simulink model "final_proj_part_d"  (R2023b)
settings: Solver=ode45  StartTime=0.0  StopTime=10  RelTol=1e-3  EnableMultiTasking=on
libraries: roblocks x2
settings Model: Creator=Chris  LastModifiedBy=kangwang
settings SolverCC: AlgebraicLoopSolver=TrustRegion
settings DataIOCC: LimitDataPoints=on  SaveFormat=Array  SignalLoggingSaveFormat=ModelDataLogs  ReturnWorkspaceOutputs=off
settings OptimizationCC: InitFltsAndDblsToZero=on  LifeSpan=inf
settings DebuggingCC: SaveWithParameterizedLinksMsg=none  UnderspecifiedInitializationDetection=Classic  MergeDetectMultiDrivingBlocksExec=none  SignalResolutionControl=TryResolveAllWithWarning  SolverPrmCheckMsg=warning  MultiTaskDSMMsg=warning  MultiTaskCondExecSysMsg=none  UnconnectedInputMsg=warning  UnconnectedOutputMsg=warning  UnconnectedLineMsg=warning  SFUnexpectedBacktrackingDiag=warning  SFNoUnconditionalDefaultTransitionDiag=warning  SFExecutionAtInitializationDiag=none  ArithmeticOperatorsInVariantConditions=warning
settings HardwareCC: ProdBitPerPointer=32  ProdBitPerSizeT=32  ProdBitPerPtrDiffT=32  ProdLargestAtomicFloat=None  ProdIntDivRoundTo=Undefined  ProdEndianess=Unspecified  ProdWordSize=32  ProdHWDeviceType=32-bit Generic
settings ModelReferenceCC: PropagateSignalLabelsOutOfModel=off
settings SFSimCC: SimUseLocalCustomCode=off  CustomCodeUndefinedFunction=UseInterfaceOnly
settings RTWCC: RTWUseLocalCustomCode=off
settings CodeAppCC: StateflowObjectComments=on
settings GRTTargetCC: TargetFcnLib=ansi_tfl_tmw.mat  TargetLangStandard=C89/C90 (ANSI)  CombineOutputUpdateFcns=off  GRTInterface=on
settings ConfigComp: CovMetricSettings=dw  CovSaveCumulativeToWorkspaceVar=on  CovSaveSingleToWorkspaceVar=on  CovExternalEMLEnable=off

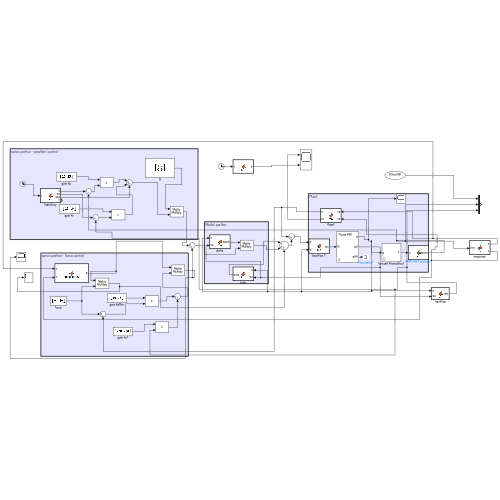
[thumbnail: Simulink's stored preview of the top-level diagram]
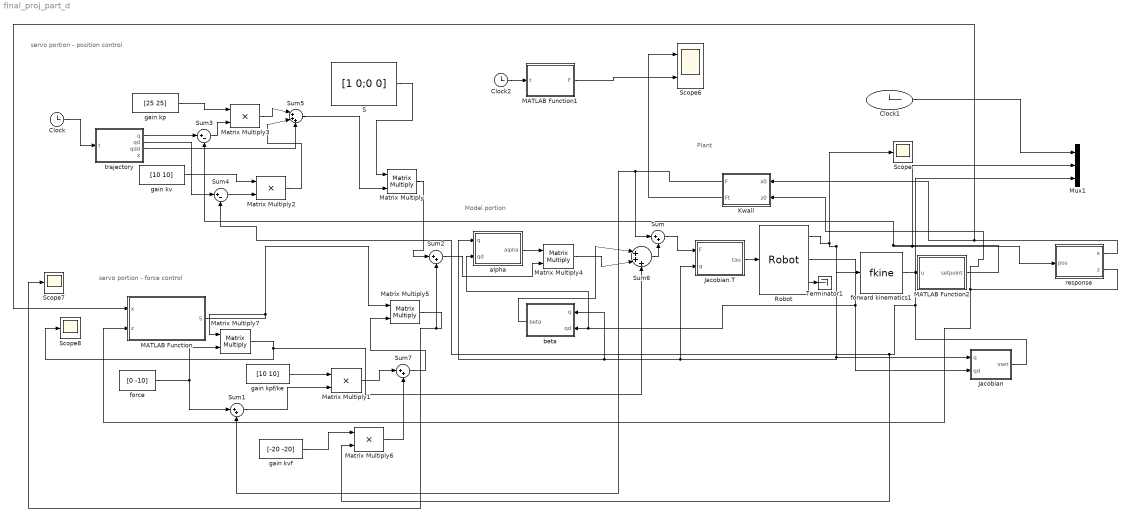
== system final_proj_part_d ==
  note: servo portion - force control
  note: Model portion
  note: Plant
  note: servo portion - position control
  Clock : Clock
  Clock1 : Clock
  Clock2 : Clock
  Jacobian : MATLAB Function  TreatAsAtomicUnit=on
  "Jacobian.T " : MATLAB Function  TreatAsAtomicUnit=on
  Kwall : MATLAB Function  TreatAsAtomicUnit=on
  MATLAB Function : MATLAB Function  TreatAsAtomicUnit=on
  MATLAB Function1 : MATLAB Function  TreatAsAtomicUnit=on
  MATLAB Function2 : MATLAB Function  TreatAsAtomicUnit=on
  Matrix Multiply{,4..5,7} (4 alike) : Product  Multiplication=Matrix(*)
  Matrix Multiply{1..3,6} (4 alike) : Product
  Mux1 : Mux  Inputs=3
  Robot : roblocks/Arm/Robot  robot=p560  q0=qn
  S : Constant  Value=[1 0;0 0]
  Scope : Scope
  Scope6 : Scope  NumInputPorts=2
  Scope7 : Scope
  Scope8 : Scope
  Sum{,1..2,7} (4 alike) : Sum  Inputs=|++
  Sum3 : Sum  Inputs=|+-
  Sum4 : Sum  Inputs=|+-
  Sum5 : Sum  Inputs=|+++
  Sum6 : Sum  Inputs=|+++
  Terminator1 : Terminator
  alpha : MATLAB Function  TreatAsAtomicUnit=on
  beta : MATLAB Function  TreatAsAtomicUnit=on
  force : Constant  Value=[0 -10]
  forward kinematics1 : roblocks/Arm/fkine  robot=robot
  gain kp : Constant  Value=[25 25]
  gain kpf/ke : Constant  Value=[10 10]
  gain kv : Constant  Value=[10 10]
  gain kvf : Constant  Value=[-20 -20]
  response : MATLAB Function  TreatAsAtomicUnit=on
  trajectory : MATLAB Function  TreatAsAtomicUnit=on
  wires:
  beta/1(beta) -> Sum6/1
  gain kp/1 -> Matrix Multiply3/1
  Matrix Multiply2/1 -> Sum5/2
  Matrix Multiply3/1 -> Sum5/1
  Matrix Multiply4/1 -> Sum6/2
  Robot/1 -> forward kinematics1/1, alpha/1(q), beta/1(q), "Jacobian.T "/2(q), Jacobian/1(q), Scope/1
  Sum3/1 -> Matrix Multiply3/2
  alpha/1(alpha) -> Matrix Multiply4/1
  Sum4/1 -> Matrix Multiply2/2
  gain kv/1 -> Matrix Multiply2/1
  Robot/3 -> Terminator1/1
  Clock1/1 -> Mux1/1
  MATLAB Function2/1(setpoint) -> Sum3/2, Mux1/2, response/1(pos)
  Robot/2 -> alpha/2(qd), beta/2(qd), Jacobian/2(qd)
  Jacobian/1(vset) -> Matrix Multiply6/2, Sum4/2, Mux1/3
  "Jacobian.T "/1(tau) -> Robot/1
  response/1(x) -> MATLAB Function/1(x), Kwall/1(x0)
  response/2(z) -> Kwall/2(z0), MATLAB Function/2(z)
  trajectory/1(q) -> Sum3/1
  trajectory/2(qd) -> Sum4/1
  trajectory/3(qdd) -> Sum5/3
  Clock/1 -> trajectory/1(t)
  gain kpf/ke/1 -> Matrix Multiply1/1
  gain kvf/1 -> Matrix Multiply6/1
  force/1 -> Matrix Multiply7/2, Sum1/1
  Sum1/1 -> Matrix Multiply1/2
  Kwall/1(F) -> Sum/1, Sum1/2
  Matrix Multiply1/1 -> Sum7/1
  Matrix Multiply6/1 -> Sum7/2
  Sum7/1 -> Matrix Multiply5/2
  S/1 -> Matrix Multiply/1
  Sum5/1 -> Matrix Multiply/2
  Matrix Multiply/1 -> Sum2/1
  Matrix Multiply5/1 -> Scope7/1, Sum2/2
  Sum2/1 -> Matrix Multiply4/2
  Matrix Multiply7/1 -> Scope8/1, Sum6/3
  Sum/1 -> "Jacobian.T "/1(F)
  Kwall/2(Ft) -> Scope6/1
  MATLAB Function/1(S) -> Matrix Multiply5/1, Matrix Multiply7/1
  Sum6/1 -> Sum/2
  Clock2/1 -> MATLAB Function1/1(t)
  MATLAB Function1/1(F) -> Scope6/2
  forward kinematics1/1 -> MATLAB Function2/1(u)

== matlab function final_proj_part_d/MATLAB Function ==
  data: x input; S output; z input
function S = modified_S(x, z)
if x<0.75&&z<0
    S = [0 0;0 1];
else
    S = [0 0.5;0 0.866];
end

== matlab function final_proj_part_d/response ==
  data: x output; pos input; z output
function [x, z]= fcn(pos)
x = pos(1);
z = pos(2);

== matlab function final_proj_part_d/trajectory ==
  data: t input; q output; qd output; qdd output; x output
function [q, qd, qdd, x]= fcn(t)
q = [0.5*sin(0.4*pi*t)+1; 0.25];
qd = [0.2*pi*cos(1.26*t); 0];
qdd = [0;0];
x = 0.5*sin(0.4*pi*t)+1;

== matlab function final_proj_part_d/alpha ==
  data: q input; alpha output; qd input
function alpha = fcn(q, qd)
t1 = q(1);
t2 = q(2);
dt1 = qd(1);
dt2 = qd(2);
M = [9+6*cos(t2) 3+3*cos(t2);
    3+3*cos(t2) 3];
J = [-sin(t1)-sin(t1+t2) -sin(t1+t2);
    cos(t1)+cos(t1+t2) cos(t1+t2)];
dJ = [-cos(t1)*dt1-cos(t1+t2)*(dt1+dt2) -cos(t1+t2)*(dt1+dt2);
    -sin(t1)*dt1-sin(t1+t2)*(dt1+dt2) -sin(t1+t2)*(dt1+dt2)];
Mx = inv(J.')*M*inv(J);
alpha = Mx;

== matlab function final_proj_part_d/Jacobian.T  ==
  data: F input; tau output; q input
function tau = fcn(F, q)
t1 = q(1);
t2 = q(2);
J = [-sin(t1)-sin(t1+t2) -sin(t1+t2);
    cos(t1)+cos(t1+t2) cos(t1+t2)];
J_tran = J.';
tau = J_tran*F;

== matlab function final_proj_part_d/Kwall ==
  data: x0 input; F output; z0 input; Ft output
function [F,Ft]= fcn(x0, z0)
F = [0;0];
kenv = -1000;
Ft = 0;
slope = sin(deg2rad(30))/cos(deg2rad(30));
c = slope*0.75;
a = -slope;
b = 1;
num = a*x0+b*z0+c;
den = sqrt(a^2+b^2);
dist = num/den;

if dist < 0 
    Ft = dist*kenv;
    Fz = cos(deg2rad(30))*Ft;
    Fx = sin(deg2rad(30))*Ft;
    F = [Fx; Fz];
end
if z0 < 0 && x0<0.75
    F = [0; z0*kenv];
    Ft = z0*kenv;
end

== matlab function final_proj_part_d/beta ==
  data: q input; beta output; qd input
function beta = fcn(q, qd)
t1 = q(1);
t2 = q(2);
dt1 = qd(1);
dt2 = qd(2);
V = [-3*sin(t2)*dt2^2-6*sin(t2)*dt1*dt2; 
    3*sin(t2)*dt1^2];
F = [3;3];
M = [9+6*cos(t2) 3+3*cos(t2);
    3+3*cos(t2) 3];
g = 9.81;
G = [3*g*cos(t1+t2)+6*g*cos(t1);
    3*g*cos(t1+t2)];
J = [-sin(t1)-sin(t1+t2) -sin(t1+t2);
    cos(t1)+cos(t1+t2) cos(t1+t2)];
dJ = [-cos(t1)*dt1-cos(t1+t2)*(dt1+dt2) -cos(t1+t2)*(dt1+dt2);
    -sin(t1)*dt1-sin(t1+t2)*(dt1+dt2) -sin(t1+t2)*(dt1+dt2)];
Vx = inv(J.')*(V-M*inv(J)*dJ*[dt1;dt2]);
Gx = inv(J.')*G;

%remember to multiply qd by J before timing Fx
xd = J*qd;
Fx = inv(J.')*F.*xd;
beta = Vx+Gx+Fx;

== matlab function final_proj_part_d/Jacobian ==
  data: q input; vset output; qd input
function vset = fcn(q,qd)
t1 = q(1);
t2 = q(2);
J = [-sin(t1)-sin(t1+t2) -sin(t1+t2);
    cos(t1)+cos(t1+t2) cos(t1+t2)];
pd = J*qd;
xd = pd(1);
yd = pd(2);
vset = [xd;yd];

== matlab function final_proj_part_d/MATLAB Function1 ==
  data: t input; F output
function F = fcn(t)
F =10;

== matlab function final_proj_part_d/MATLAB Function2 ==
  data: u input; setpoint output
function setpoint= fcn(u)

x = u(1,4);
y = u(2,4);
setpoint = [x;y];
